simulink model "AllModes"  (R2022a)
settings: Solver=FixedStepAuto  StartTime=0.0  StopTime=10.0  FixedStep=1e-3  RelTol=1e-3  EnableMultiTasking=on
undefined symbols (not defined in the file): D0, D1, D10, D11, D12, D13, D2, D3, D4, D5, D6, D7, D8, D9, PTA0, PTA1, PTA2, PTB23, PTB9, PTC16, PTC17, PTC2, PTC3, PTC4, PTD0, PTD1, PTD2, PTD3
libraries: frdmk64flib x14
settings Model: ExtModeTrigDuration=5  Creator=bmile  LastModifiedBy=Motz
settings OptimizationCC: EnhancedBackFolding=on  PassReuseOutputArgsAs=Individual arguments  ZeroExternalMemoryAtStartup=off  ZeroInternalMemoryAtStartup=off  MaxStackSize=64  OptimizeBlockOrder=speed  DifferentSizesBufferReuse=on  OptimizationCustomize=off  EfficientTunableParamExpr=on
settings DebuggingCC: ParameterTunabilityLossMsg=error
settings HardwareCC: ProdBitPerPointer=32  ProdBitPerSizeT=32  ProdBitPerPtrDiffT=32  ProdLargestAtomicInteger=Long  ProdLargestAtomicFloat=Double  ProdWordSize=32  ProdHWDeviceType=ARM Compatible->ARM Cortex
settings SFSimCC: MATLABDynamicMemAlloc=off
settings RTWCC: SystemTargetFile=ert.tlc  HardwareBoard=NXP FRDM-K64F  TLCOptions="-aInlineSetEventsForThisBaseRateFcn=TLC_FALSE -aSuppressMultiTaskScheduler=TLC_FALSE  -aRateBasedStepFcn=0"  TemplateMakefile=ert_default_tmf  Toolchain=GNU Tools for ARM Embedded Processors
settings CodeAppCC: ForceParamTrailComments=on  IgnoreCustomStorageClasses=off  OperatorAnnotations=on  SimulinkDataObjDesc=on  SFDataObjDesc=on  InsertBlockDesc=on
settings ERTTargetCC: ExtModeTransport=4  ExtModeMexFile=sendToCommService

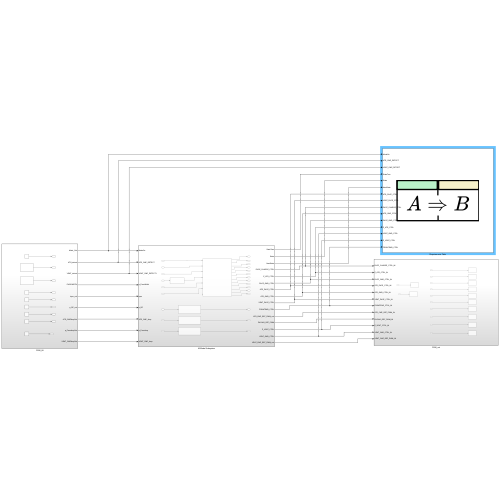
[thumbnail: Simulink's stored preview of the top-level diagram]
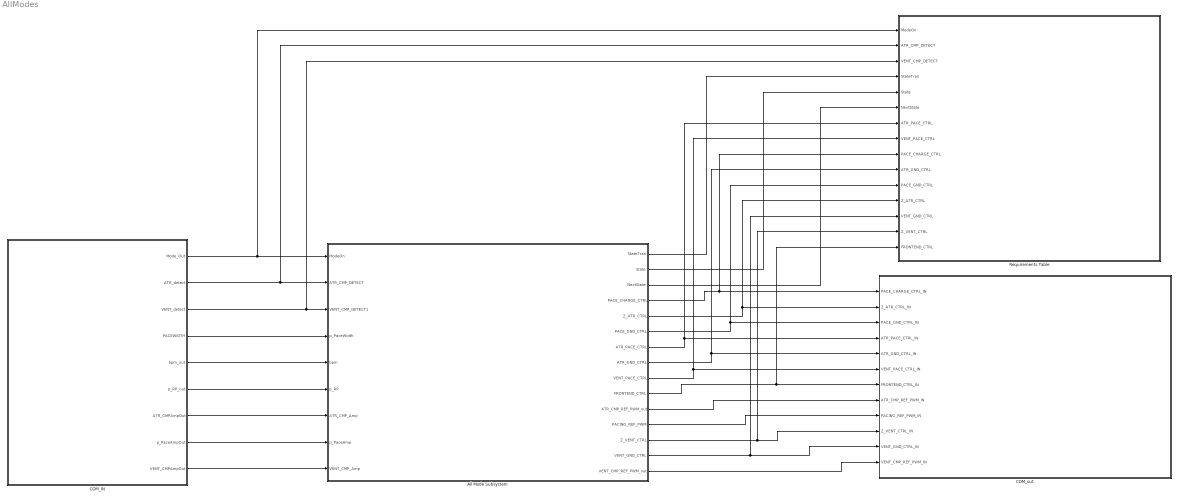
== system AllModes ==
  All Mode Subsystem : Subsystem
  COM_IN : Subsystem
  COM_out : Subsystem
  Requirements Table : Requirements Table  TreatAsAtomicUnit=on
  wires:
  COM_IN/1(Mode_Out) -> All Mode Subsystem/1(ModeOn), Requirements Table/1(ModeOn)
  COM_IN/4(PACEWIDTH) -> All Mode Subsystem/4(p_PaceWidth)
  COM_IN/5(bpm_out) -> All Mode Subsystem/5(bpm)
  COM_IN/6(p_RP_out) -> All Mode Subsystem/6(p_RP)
  COM_IN/7(ATR_CMPAmpOut) -> All Mode Subsystem/7(ATR_CMP_Amp)
  COM_IN/8(p_PaceAmpOut) -> All Mode Subsystem/8(p_PaceAmp)
  COM_IN/9(VENT_CMPAmpOut) -> All Mode Subsystem/9(VENT_CMP_Amp)
  All Mode Subsystem/4(PACE_CHARGE_CTRL) -> Requirements Table/9(PACE_CHARGE_CTRL), COM_out/1(PACE_CHARGE_CTRL_IN)
  All Mode Subsystem/5(Z_ATR_CTRL) -> Requirements Table/12(Z_ATR_CTRL), COM_out/2(Z_ATR_CTRL_IN)
  All Mode Subsystem/6(PACE_GND_CTRL) -> Requirements Table/11(PACE_GND_CTRL), COM_out/3(PACE_GND_CTRL_IN)
  All Mode Subsystem/7(ATR_PACE_CTRL) -> Requirements Table/7(ATR_PACE_CTRL), COM_out/4(ATR_PACE_CTRL_IN)
  All Mode Subsystem/9(VENT_PACE_CTRL) -> Requirements Table/8(VENT_PACE_CTRL), COM_out/6(VENT_PACE_CTRL_IN)
  All Mode Subsystem/10(FRONTEND_CTRL) -> Requirements Table/15(FRONTEND_CTRL), COM_out/7(FRONTEND_CTRL_IN)
  All Mode Subsystem/11(ATR_CMP_REF_PWM_out) -> COM_out/8(ATR_CMP_REF_PWM_IN)
  All Mode Subsystem/12(PACING_REF_PWM) -> COM_out/9(PACING_REF_PWM_IN)
  All Mode Subsystem/13(Z_VENT_CTRL) -> Requirements Table/14(Z_VENT_CTRL), COM_out/10(Z_VENT_CTRL_IN)
  All Mode Subsystem/14(VENT_GND_CTRL) -> Requirements Table/13(VENT_GND_CTRL), COM_out/11(VENT_GND_CTRL_IN)
  All Mode Subsystem/15(VENT_CMP_REF_PWM_out) -> COM_out/12(VENT_CMP_REF_PWM_IN)
  All Mode Subsystem/3(NextState) -> Requirements Table/6(NextState)
  All Mode Subsystem/2(State) -> Requirements Table/5(State)
  All Mode Subsystem/8(ATR_GND_CTRL) -> Requirements Table/10(ATR_GND_CTRL), COM_out/5(ATR_GND_CTRL_IN)
  All Mode Subsystem/1(StateTran) -> Requirements Table/4(StateTran)
  COM_IN/2(ATR_detect) -> All Mode Subsystem/2(ATR_CMP_DETECT), Requirements Table/2(ATR_CMP_DETECT)
  COM_IN/3(VENT_detect) -> Requirements Table/3(VENT_CMP_DETECT), All Mode Subsystem/3(VENT_CMP_DETECT1)

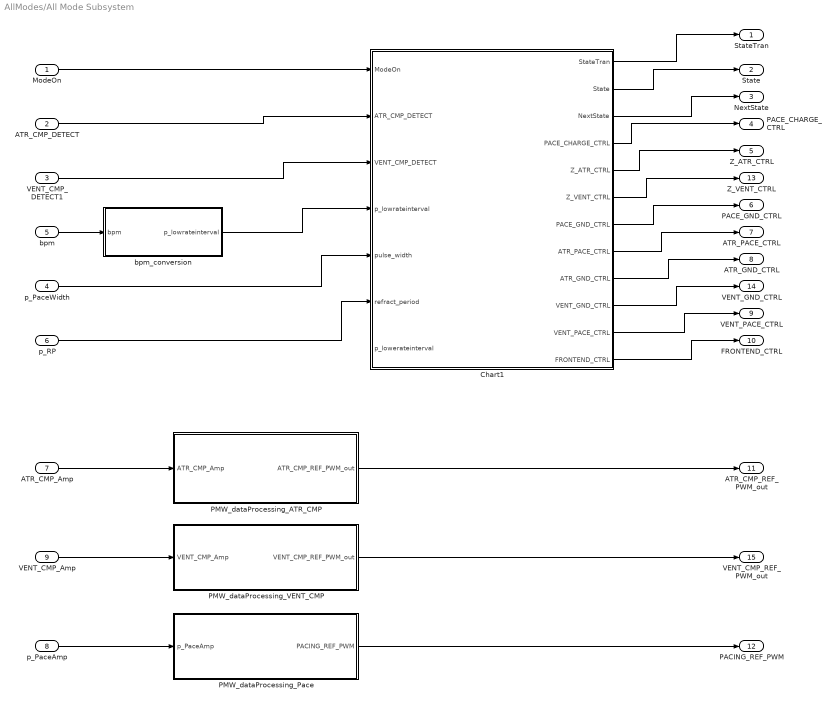
== system AllModes/All Mode Subsystem ==
  ModeOn : Inport
  ATR_CMP_DETECT : Inport  Port=2
  VENT_CMP_DETECT1 : Inport  Port=3
  p_PaceWidth : Inport  Port=4
  bpm : Inport  Port=5
  p_RP : Inport  Port=6
  ATR_CMP_Amp : Inport  Port=7
  p_PaceAmp : Inport  Port=8
  VENT_CMP_Amp : Inport  Port=9
  Chart1 : Stateflow chart  TreatAsAtomicUnit=on
      settings: PortSchema="{\"entries\":[{\"content\":{\"sides\":[{\"content\":{\"connectorIds\":[\"In1\",\"In2\",\"In3\",\"In4\",\"In5\",\"In6\",\"In7\"]},\"type\":\"ConnectorPlacement.EquallySpacedRectSide\",\"uuid\":\"7ea964f2-2529-4e69-b20d-c2fa6008c3a7\"},{\"content\":{\"connectorIds\":[\"Out12\",\"Out1\",\"Out11\",\"Out2\",\"Out3\",\"Out4\",\"Out5\",\"Out6\",\"Out7\",\"Out8\",\"Out9\",\"Out10\"],\"side\":\"RIGHT\"},\"type\":\"ConnectorPlacement.EquallySpacedRectSide\",\"uuid\":\"c561387b-bc02-43ab-893b-c9cb757a1c6a\"},{\"content\":{\"connectorIds\":[],\"side\":\"TOP\"},\"type\":\"ConnectorPlacement.EquallySpacedRectSide\",\"uuid\":\"1f667392-9a0f-4cad-82e3-6fe4d50b6af4\"}]},\"type\":\"ConnectorPlacement.EquallySpacedConnector\",\"uuid\":\"bd362c40-ffc0-452d-8626-3f1602423ca2\"}],\"packageUris\":[\"http://schema.mathworks.com/mf0/Connector/R2020b\"],\"version\":\"1.0\"}"
  PMW_dataProcessing_ATR_CMP : Subsystem
  PMW_dataProcessing_Pace : Subsystem
  PMW_dataProcessing_VENT_CMP : Subsystem
  bpm_conversion : Subsystem
  StateTran : Outport
  State : Outport  Port=2
  NextState : Outport  Port=3
  PACE_CHARGE_CTRL : Outport  Port=4
  Z_ATR_CTRL : Outport  Port=5
  PACE_GND_CTRL : Outport  Port=6
  ATR_PACE_CTRL : Outport  Port=7
  ATR_GND_CTRL : Outport  Port=8
  VENT_PACE_CTRL : Outport  Port=9
  FRONTEND_CTRL : Outport  Port=10
  ATR_CMP_REF_PWM_out : Outport  Port=11
  PACING_REF_PWM : Outport  Port=12
  Z_VENT_CTRL : Outport  Port=13
  VENT_GND_CTRL : Outport  Port=14
  VENT_CMP_REF_PWM_out : Outport  Port=15
  wires:
  Chart1/10(FRONTEND_CTRL) -> FRONTEND_CTRL/1
  Chart1/9(VENT_PACE_CTRL) -> VENT_PACE_CTRL/1
  Chart1/7(ATR_GND_CTRL) -> ATR_GND_CTRL/1
  Chart1/6(ATR_PACE_CTRL) -> ATR_PACE_CTRL/1
  Chart1/5(PACE_GND_CTRL) -> PACE_GND_CTRL/1
  Chart1/3(Z_ATR_CTRL) -> Z_ATR_CTRL/1
  Chart1/2(PACE_CHARGE_CTRL) -> PACE_CHARGE_CTRL/1
  p_RP/1 -> Chart1/6(refract_period)
  p_PaceWidth/1 -> Chart1/5(pulse_width)
  ATR_CMP_DETECT/1 -> Chart1/2(ATR_CMP_DETECT)
  Chart1/1(State) -> State/1
  ModeOn/1 -> Chart1/1(ModeOn)
  Chart1/4(Z_VENT_CTRL) -> Z_VENT_CTRL/1
  Chart1/8(VENT_GND_CTRL) -> VENT_GND_CTRL/1
  VENT_CMP_DETECT1/1 -> Chart1/3(VENT_CMP_DETECT)
  ATR_CMP_Amp/1 -> PMW_dataProcessing_ATR_CMP/1(ATR_CMP_Amp)
  p_PaceAmp/1 -> PMW_dataProcessing_Pace/1(p_PaceAmp)
  VENT_CMP_Amp/1 -> PMW_dataProcessing_VENT_CMP/1(VENT_CMP_Amp)
  PMW_dataProcessing_Pace/1(PACING_REF_PWM) -> PACING_REF_PWM/1
  PMW_dataProcessing_VENT_CMP/1(VENT_CMP_REF_PWM_out) -> VENT_CMP_REF_PWM_out/1
  PMW_dataProcessing_ATR_CMP/1(ATR_CMP_REF_PWM_out) -> ATR_CMP_REF_PWM_out/1
  bpm/1 -> bpm_conversion/1(bpm)
  bpm_conversion/1(p_lowrateinterval) -> Chart1/4(p_lowrateinterval)
  Chart1/11(NextState) -> NextState/1
  Chart1/12(StateTran) -> StateTran/1

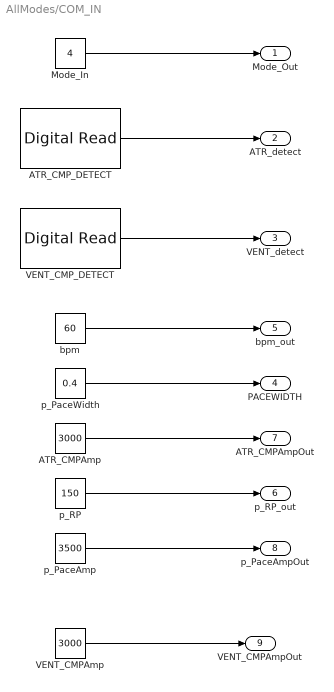
== system AllModes/COM_IN ==
  ATR_CMPAmp : Constant  Value=3000
  ATR_CMP_DETECT : frdmk64flib/Digital Read  Whichpin=PTC16 (D0)  SampleTime=-1
  Mode_In : Constant  Value=4
  VENT_CMPAmp : Constant  Value=3000
  VENT_CMP_DETECT : frdmk64flib/Digital Read  Whichpin=PTC17 (D1)  SampleTime=-1
  bpm : Constant  Value=60
  p_PaceAmp : Constant  Value=3500
  p_PaceWidth : Constant  Value=0.4
  p_RP : Constant  Value=150
  Mode_Out : Outport
  ATR_detect : Outport  Port=2
  VENT_detect : Outport  Port=3
  PACEWIDTH : Outport  Port=4
  bpm_out : Outport  Port=5
  p_RP_out : Outport  Port=6
  ATR_CMPAmpOut : Outport  Port=7
  p_PaceAmpOut : Outport  Port=8
  VENT_CMPAmpOut : Outport  Port=9
  wires:
  Mode_In/1 -> Mode_Out/1
  ATR_CMP_DETECT/1 -> ATR_detect/1
  bpm/1 -> bpm_out/1
  ATR_CMPAmp/1 -> ATR_CMPAmpOut/1
  VENT_CMP_DETECT/1 -> VENT_detect/1
  p_PaceWidth/1 -> PACEWIDTH/1
  p_RP/1 -> p_RP_out/1
  p_PaceAmp/1 -> p_PaceAmpOut/1
  VENT_CMPAmp/1 -> VENT_CMPAmpOut/1

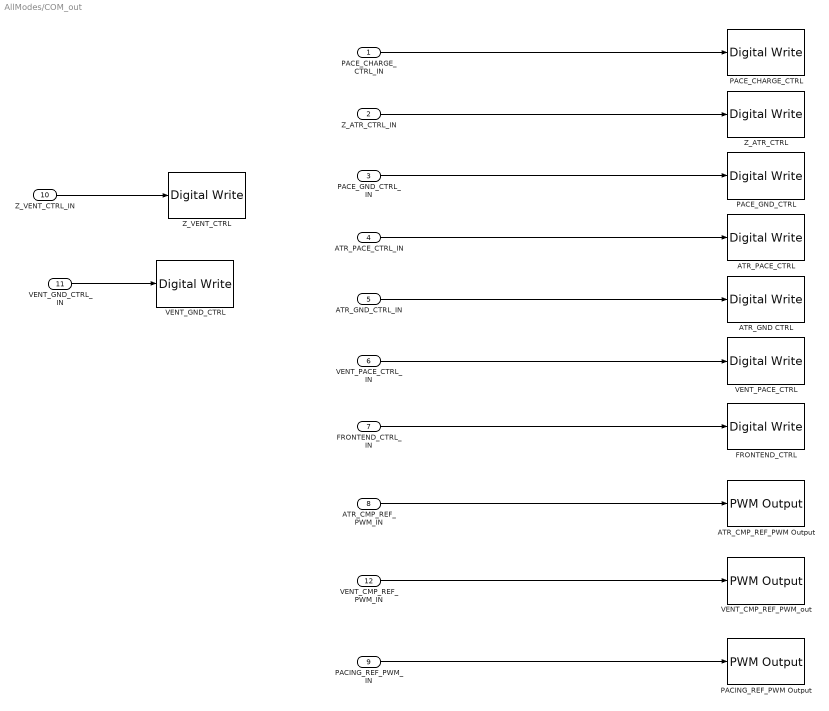
== system AllModes/COM_out ==
  PACE_CHARGE_CTRL_IN : Inport
  Z_ATR_CTRL_IN : Inport  Port=2
  PACE_GND_CTRL_IN : Inport  Port=3
  ATR_PACE_CTRL_IN : Inport  Port=4
  ATR_GND_CTRL_IN : Inport  Port=5
  VENT_PACE_CTRL_IN : Inport  Port=6
  FRONTEND_CTRL_IN : Inport  Port=7
  ATR_CMP_REF_PWM_IN : Inport  Port=8
  PACING_REF_PWM_IN : Inport  Port=9
  Z_VENT_CTRL_IN : Inport  Port=10
  VENT_GND_CTRL_IN : Inport  Port=11
  VENT_CMP_REF_PWM_IN : Inport  Port=12
  ATR_CMP_REF_PWM Output : frdmk64flib/PWM Output  Whichpin=PTC2 (D6)  InitialFrequency=2000  InitialDutyCycle=0
  ATR_GND CTRL : frdmk64flib/Digital Write  Whichpin=PTD2 (D11)
  ATR_PACE_CTRL : frdmk64flib/Digital Write  Whichpin=PTA0 (D8)
  FRONTEND_CTRL : frdmk64flib/Digital Write  Whichpin=PTD1 (D13)
  PACE_CHARGE_CTRL : frdmk64flib/Digital Write  Whichpin=PTB9 (D2)
  PACE_GND_CTRL : frdmk64flib/Digital Write  Whichpin=PTD0 (D10)
  PACING_REF_PWM Output : frdmk64flib/PWM Output  Whichpin=PTA2 (D5)  InitialFrequency=2000  InitialDutyCycle=0
  VENT_CMP_REF_PWM_out : frdmk64flib/PWM Output  Whichpin=PTA1 (D3)  InitialFrequency=2000  InitialDutyCycle=0
  VENT_GND_CTRL : frdmk64flib/Digital Write  Whichpin=PTD3 (D12)
  VENT_PACE_CTRL : frdmk64flib/Digital Write  Whichpin=PTC4 (D9)
  Z_ATR_CTRL : frdmk64flib/Digital Write  Whichpin=PTB23 (D4)
  Z_VENT_CTRL : frdmk64flib/Digital Write  Whichpin=PTC3 (D7)
  wires:
  PACE_CHARGE_CTRL_IN/1 -> PACE_CHARGE_CTRL/1
  PACE_GND_CTRL_IN/1 -> PACE_GND_CTRL/1
  Z_ATR_CTRL_IN/1 -> Z_ATR_CTRL/1
  ATR_PACE_CTRL_IN/1 -> ATR_PACE_CTRL/1
  ATR_GND_CTRL_IN/1 -> ATR_GND CTRL/1
  VENT_PACE_CTRL_IN/1 -> VENT_PACE_CTRL/1
  FRONTEND_CTRL_IN/1 -> FRONTEND_CTRL/1
  PACING_REF_PWM_IN/1 -> PACING_REF_PWM Output/1
  ATR_CMP_REF_PWM_IN/1 -> ATR_CMP_REF_PWM Output/1
  VENT_GND_CTRL_IN/1 -> VENT_GND_CTRL/1
  Z_VENT_CTRL_IN/1 -> Z_VENT_CTRL/1
  VENT_CMP_REF_PWM_IN/1 -> VENT_CMP_REF_PWM_out/1

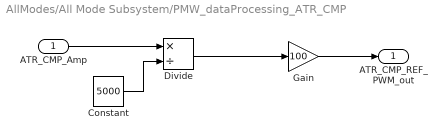
== system AllModes/All Mode Subsystem/PMW_dataProcessing_ATR_CMP ==
  ATR_CMP_Amp : Inport
  Constant : Constant  Value=5000
  Divide : Product  Inputs=*/
  Gain : Gain  Gain=100
  ATR_CMP_REF_PWM_out : Outport
  wires:
  Divide/1 -> Gain/1
  Constant/1 -> Divide/2
  ATR_CMP_Amp/1 -> Divide/1
  Gain/1 -> ATR_CMP_REF_PWM_out/1

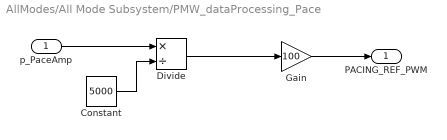
== system AllModes/All Mode Subsystem/PMW_dataProcessing_Pace ==
  p_PaceAmp : Inport
  Constant : Constant  Value=5000
  Divide : Product  Inputs=*/
  Gain : Gain  Gain=100
  PACING_REF_PWM : Outport
  wires:
  Divide/1 -> Gain/1
  Constant/1 -> Divide/2
  p_PaceAmp/1 -> Divide/1
  Gain/1 -> PACING_REF_PWM/1

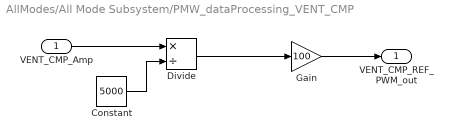
== system AllModes/All Mode Subsystem/PMW_dataProcessing_VENT_CMP ==
  VENT_CMP_Amp : Inport
  Constant : Constant  Value=5000
  Divide : Product  Inputs=*/
  Gain : Gain  Gain=100
  VENT_CMP_REF_PWM_out : Outport
  wires:
  Divide/1 -> Gain/1
  Constant/1 -> Divide/2
  VENT_CMP_Amp/1 -> Divide/1
  Gain/1 -> VENT_CMP_REF_PWM_out/1

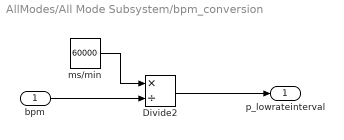
== system AllModes/All Mode Subsystem/bpm_conversion ==
  bpm : Inport
  Divide2 : Product  Inputs=*/
  ms/min : Constant  Value=60000
  p_lowrateinterval : Outport
  wires:
  ms/min/1 -> Divide2/1
  bpm/1 -> Divide2/2
  Divide2/1 -> p_lowrateinterval/1

== stateflow chart AllModes/Requirements Table ==
  (default) -> (junction 1073742992)
  (junction 1073742992) -> (junction 1073742993) : {
      | % SF_REQ_REV_07
      | }
  (junction 1073742993) -> (junction 1073742995) : {
      | % HEADER_ASSIGNMENTS
      |
      | }
  (junction 1073742995) -> (junction 1073742997) : {
      | % START_A_4
      | }
  (junction 1073742997) -> (junction 1073742999) : {
      | }
  (junction 1073742999) -> (junction 1073743001)
  (junction 1073743001) -> (junction 1073743003) : {
      | }
  (junction 1073743003) -> (junction 1073743005) : {
      | % END_A_4
      | }
  (junction 1073743005) -> (junction 1073743007) : {
      | % START_R_7
      | }
  (junction 1073743007) -> (junction 1073743009) : {
      | }
  (junction 1073743009) -> (junction 1073743011)
  (junction 1073743011) -> (junction 1073743013) [order 1] : [(((State) == (0)))]
  (junction 1073743011) -> (junction 1073743091) [order 2]
  (junction 1073743013) -> (junction 1073743015) : {
      | reqtable_postcondition((((NextState) == (0))) && (((ATR_PACE_CTRL) == (false))) && (((VENT_PACE_CTRL) == (false))) && (((PACE_CHARGE_CTRL) == (false))) && (((ATR_GND_CTRL) == (false))) && (((PACE_GND_CTRL) == (false))) && (((Z_ATR_CTRL) == (false))) && (((VENT_GND_CTRL) == (false))) && (((Z_VENT_CTRL) == (false))) && (((FRONTEND_CTRL) == (false))), 'R:1');
      |
      |
      | }
  (junction 1073743015) -> (junction 1073743017) : {
      | }
  (junction 1073743017) -> (junction 1073743019) : {
      | % START_R_10
      | }
  (junction 1073743019) -> (junction 1073743021) : {
      | }
  (junction 1073743021) -> (junction 1073743023)
  (junction 1073743023) -> (junction 1073743025) [order 1] : [(((StateTran) == (true))) && (((ModeOn) == (1)))]
  (junction 1073743023) -> (junction 1073743031) [order 2]
  (junction 1073743025) -> (junction 1073743027) : {
      | reqtable_postcondition((((NextState) == (1))) && (((ATR_PACE_CTRL) == (false))) && (((VENT_PACE_CTRL) == (false))) && (((PACE_CHARGE_CTRL) == (false))) && (((ATR_GND_CTRL) == (false))) && (((PACE_GND_CTRL) == (false))) && (((Z_ATR_CTRL) == (false))) && (((VENT_GND_CTRL) == (false))) && (((Z_VENT_CTRL) == (false))) && (((FRONTEND_CTRL) == (false))), 'R:1.1');
      |
      |
      | }
  (junction 1073743027) -> (junction 1073743029) : {
      | }
  (junction 1073743029) -> (junction 1073743031)
  (junction 1073743031) -> (junction 1073743033)
  (junction 1073743033) -> (junction 1073743035) : {
      | % END_R_10
      | }
  (junction 1073743035) -> (junction 1073743037) : {
      | % START_R_16
      | }
  (junction 1073743037) -> (junction 1073743039) : {
      | }
  (junction 1073743039) -> (junction 1073743041)
  (junction 1073743041) -> (junction 1073743043) [order 1] : [(((StateTran) == (true))) && (((ModeOn) == (2)))]
  (junction 1073743041) -> (junction 1073743049) [order 2]
  (junction 1073743043) -> (junction 1073743045) : {
      | reqtable_postcondition((((NextState) == (2))) && (((ATR_PACE_CTRL) == (false))) && (((VENT_PACE_CTRL) == (false))) && (((PACE_CHARGE_CTRL) == (false))) && (((ATR_GND_CTRL) == (false))) && (((PACE_GND_CTRL) == (false))) && (((Z_ATR_CTRL) == (false))) && (((VENT_GND_CTRL) == (false))) && (((Z_VENT_CTRL) == (false))) && (((FRONTEND_CTRL) == (false))), 'R:1.2');
      |
      |
      | }
  (junction 1073743045) -> (junction 1073743047) : {
      | }
  (junction 1073743047) -> (junction 1073743049)
  (junction 1073743049) -> (junction 1073743051)
  (junction 1073743051) -> (junction 1073743053) : {
      | % END_R_16
      | }
  (junction 1073743053) -> (junction 1073743055) : {
      | % START_R_19
      | }
  (junction 1073743055) -> (junction 1073743057) : {
      | }
  (junction 1073743057) -> (junction 1073743059)
  (junction 1073743059) -> (junction 1073743061) [order 1] : [(((StateTran) == (true))) && (((ModeOn) == (3)))]
  (junction 1073743059) -> (junction 1073743067) [order 2]
  (junction 1073743061) -> (junction 1073743063) : {
      | reqtable_postcondition((((NextState) == (3))) && (((ATR_PACE_CTRL) == (false))) && (((VENT_PACE_CTRL) == (false))) && (((PACE_CHARGE_CTRL) == (false))) && (((ATR_GND_CTRL) == (false))) && (((PACE_GND_CTRL) == (false))) && (((Z_ATR_CTRL) == (false))) && (((VENT_GND_CTRL) == (false))) && (((Z_VENT_CTRL) == (false))) && (((FRONTEND_CTRL) == (false))), 'R:1.3');
      |
      |
      | }
  (junction 1073743063) -> (junction 1073743065) : {
      | }
  (junction 1073743065) -> (junction 1073743067)
  (junction 1073743067) -> (junction 1073743069)
  (junction 1073743069) -> (junction 1073743071) : {
      | % END_R_19
      | }
  (junction 1073743071) -> (junction 1073743073) : {
      | % START_R_22
      | }
  (junction 1073743073) -> (junction 1073743075) : {
      | }
  (junction 1073743075) -> (junction 1073743077)
  (junction 1073743077) -> (junction 1073743079) [order 1] : [(((StateTran) == (true))) && (((ModeOn) == (4)))]
  (junction 1073743077) -> (junction 1073743085) [order 2]
  (junction 1073743079) -> (junction 1073743081) : {
      | reqtable_postcondition((((NextState) == (4))), 'R:1.4');
      |
      |
      | }
  (junction 1073743081) -> (junction 1073743083) : {
      | }
  (junction 1073743083) -> (junction 1073743085)
  (junction 1073743085) -> (junction 1073743087)
  (junction 1073743087) -> (junction 1073743089) : {
      | % END_R_22
      | }
  (junction 1073743089) -> (junction 1073743091)
  (junction 1073743091) -> (junction 1073743093)
  (junction 1073743093) -> (junction 1073743095) : {
      | % END_R_7
      | }
  (junction 1073743095) -> (junction 1073743097) : {
      | % START_R_1
      | }
  (junction 1073743097) -> (junction 1073743099) : {
      | }
  (junction 1073743099) -> (junction 1073743101)
  (junction 1073743101) -> (junction 1073743103) [order 1] : [(((State) == (1)))]
  (junction 1073743101) -> (junction 1073743127) [order 2]
  (junction 1073743103) -> (junction 1073743105) : {
      | reqtable_postcondition((((NextState) == (0))) && (((ATR_PACE_CTRL) == (false))) && (((VENT_PACE_CTRL) == (false))) && (((PACE_CHARGE_CTRL) == (true))) && (((ATR_GND_CTRL) == (true))) && (((PACE_GND_CTRL) == (true))) && (((Z_ATR_CTRL) == (false))) && (((VENT_GND_CTRL) == (false))) && (((Z_VENT_CTRL) == (false))) && (((FRONTEND_CTRL) == (false))), 'R:2');
      |
      |
      | }
  (junction 1073743105) -> (junction 1073743107) : {
      | }
  (junction 1073743107) -> (junction 1073743109) : {
      | % START_R_28
      | }
  (junction 1073743109) -> (junction 1073743111) : {
      | }
  (junction 1073743111) -> (junction 1073743113)
  (junction 1073743113) -> (junction 1073743115) [order 1] : [(((StateTran) == (true)))]
  (junction 1073743113) -> (junction 1073743121) [order 2]
  (junction 1073743115) -> (junction 1073743117) : {
      | reqtable_postcondition((((NextState) == (2))), 'R:2.1');
      |
      |
      | }
  (junction 1073743117) -> (junction 1073743119) : {
      | }
  (junction 1073743119) -> (junction 1073743121)
  (junction 1073743121) -> (junction 1073743123)
  (junction 1073743123) -> (junction 1073743125) : {
      | % END_R_28
      | }
  (junction 1073743125) -> (junction 1073743127)
  (junction 1073743127) -> (junction 1073743129)
  (junction 1073743129) -> (junction 1073743131) : {
      | % END_R_1
      | }
  (junction 1073743131) -> (junction 1073743133) : {
      | % START_R_25
      | }
  (junction 1073743133) -> (junction 1073743135) : {
      | }
  (junction 1073743135) -> (junction 1073743137)
  (junction 1073743137) -> (junction 1073743139) [order 1] : [(((State) == (2)))]
  (junction 1073743137) -> (junction 1073743313) [order 2]
  (junction 1073743139) -> (junction 1073743141) : {
      | reqtable_postcondition((((NextState) == (0))) && (((ATR_PACE_CTRL) == (true))) && (((VENT_PACE_CTRL) == (false))) && (((PACE_CHARGE_CTRL) == (false))) && (((ATR_GND_CTRL) == (false))) && (((PACE_GND_CTRL) == (true))) && (((Z_ATR_CTRL) == (false))) && (((VENT_GND_CTRL) == (false))) && (((Z_VENT_CTRL) == (false))) && (((FRONTEND_CTRL) == (false))), 'R:3');
      |
      |
      | }
  (junction 1073743141) -> (junction 1073743143) : {
      | }
  (junction 1073743143) -> (junction 1073743145) : {
      | % START_R_31
      | }
  (junction 1073743145) -> (junction 1073743147) : {
      | }
  (junction 1073743147) -> (junction 1073743149)
  (junction 1073743149) -> (junction 1073743151) [order 1] : [(((StateTran) == (true)))]
  (junction 1073743149) -> (junction 1073743157) [order 2]
  (junction 1073743151) -> (junction 1073743153) : {
      | reqtable_postcondition((((NextState) == (1))), 'R:3.1');
      |
      |
      | }
  (junction 1073743153) -> (junction 1073743155) : {
      | }
  (junction 1073743155) -> (junction 1073743157)
  (junction 1073743157) -> (junction 1073743159)
  (junction 1073743159) -> (junction 1073744214) : {
      | % END_R_31
      | }
  (junction 1073744214) -> (junction 1073743313)
  (junction 1073743313) -> (junction 1073743315)
  (junction 1073743315) -> (junction 1073743317) : {
      | % END_R_25
      | }
  (junction 1073743317) -> (junction 1073744220) : {
      | % START_R_34
      | }
  (junction 1073744220) -> (junction 1073744222) : {
      | }
  (junction 1073744222) -> (junction 1073744224)
  (junction 1073744224) -> (junction 1073744226) [order 1] : [(((State) == (3)))]
  (junction 1073744224) -> (junction 1073744250) [order 2]
  (junction 1073744226) -> (junction 1073744228) : {
      | reqtable_postcondition((((NextState) == (0))) && (((ATR_PACE_CTRL) == (false))) && (((VENT_PACE_CTRL) == (false))) && (((PACE_CHARGE_CTRL) == (true))) && (((ATR_GND_CTRL) == (false))) && (((PACE_GND_CTRL) == (true))) && (((Z_ATR_CTRL) == (false))) && (((VENT_GND_CTRL) == (true))) && (((Z_VENT_CTRL) == (false))) && (((FRONTEND_CTRL) == (false))), 'R:4');
      |
      |
      | }
  (junction 1073744228) -> (junction 1073744230) : {
      | }
  (junction 1073744230) -> (junction 1073744232) : {
      | % START_R_37
      | }
  (junction 1073744232) -> (junction 1073744234) : {
      | }
  (junction 1073744234) -> (junction 1073744236)
  (junction 1073744236) -> (junction 1073744238) [order 1] : [(((StateTran) == (true)))]
  (junction 1073744236) -> (junction 1073744244) [order 2]
  (junction 1073744238) -> (junction 1073744240) : {
      | reqtable_postcondition((((NextState) == (4))), 'R:4.1');
      |
      |
      | }
  (junction 1073744240) -> (junction 1073744242) : {
      | }
  (junction 1073744242) -> (junction 1073744244)
  (junction 1073744244) -> (junction 1073744246)
  (junction 1073744246) -> (junction 1073744248) : {
      | % END_R_37
      | }
  (junction 1073744248) -> (junction 1073744250)
  (junction 1073744250) -> (junction 1073744252)
  (junction 1073744252) -> (junction 1073744254) : {
      | % END_R_34
      | }
  (junction 1073744254) -> (junction 1073744260) : {
      | % START_R_43
      | }
  (junction 1073744260) -> (junction 1073744262) : {
      | }
  (junction 1073744262) -> (junction 1073744264)
  (junction 1073744264) -> (junction 1073744266) [order 1] : [(((State) == (4)))]
  (junction 1073744264) -> (junction 1073744290) [order 2]
  (junction 1073744266) -> (junction 1073744268) : {
      | reqtable_postcondition((((NextState) == (0))) && (((ATR_PACE_CTRL) == (false))) && (((VENT_PACE_CTRL) == (true))) && (((PACE_CHARGE_CTRL) == (false))) && (((ATR_GND_CTRL) == (false))) && (((PACE_GND_CTRL) == (true))) && (((Z_ATR_CTRL) == (false))) && (((VENT_GND_CTRL) == (false))) && (((Z_VENT_CTRL) == (false))) && (((FRONTEND_CTRL) == (false))), 'R:5');
      |
      |
      | }
  (junction 1073744268) -> (junction 1073744270) : {
      | }
  (junction 1073744270) -> (junction 1073744272) : {
      | % START_R_46
      | }
  (junction 1073744272) -> (junction 1073744274) : {
      | }
  (junction 1073744274) -> (junction 1073744276)
  (junction 1073744276) -> (junction 1073744278) [order 1] : [(((StateTran) == (true)))]
  (junction 1073744276) -> (junction 1073744284) [order 2]
  (junction 1073744278) -> (junction 1073744280) : {
      | reqtable_postcondition((((NextState) == (3))), 'R:5.1');
      |
      |
      | }
  (junction 1073744280) -> (junction 1073744282) : {
      | }
  (junction 1073744282) -> (junction 1073744284)
  (junction 1073744284) -> (junction 1073744286)
  (junction 1073744286) -> (junction 1073744288) : {
      | % END_R_46
      | }
  (junction 1073744288) -> (junction 1073744290)
  (junction 1073744290) -> (junction 1073744292)
  (junction 1073744292) -> (junction 1073744294) : {
      | % END_R_43
      | }
  (junction 1073744294) -> (junction 1073744121) : {
      | % START_R_49
      | }
  (junction 1073744121) -> (junction 1073744123) : {
      | }
  (junction 1073744123) -> (junction 1073744125)
  (junction 1073744125) -> (junction 1073744127) [order 1] : [(((State) == (5)))]
  (junction 1073744125) -> (junction 1073744169) [order 2]
  (junction 1073744127) -> (junction 1073744129) : {
      | reqtable_postcondition((((NextState) == (0))) && (((ATR_PACE_CTRL) == (false))) && (((VENT_PACE_CTRL) == (false))) && (((PACE_CHARGE_CTRL) == (true))) && (((ATR_GND_CTRL) == (true))) && (((PACE_GND_CTRL) == (true))) && (((Z_ATR_CTRL) == (false))) && (((VENT_GND_CTRL) == (false))) && (((Z_VENT_CTRL) == (false))) && (((FRONTEND_CTRL) == (true))), 'R:6');
      |
      |
      | }
  (junction 1073744129) -> (junction 1073744131) : {
      | }
  (junction 1073744131) -> (junction 1073744133) : {
      | % START_R_58
      | }
  (junction 1073744133) -> (junction 1073744135) : {
      | }
  (junction 1073744135) -> (junction 1073744137)
  (junction 1073744137) -> (junction 1073744139) [order 1] : [(((StateTran) == (true))) && (((ATR_CMP_DETECT) == (true)))]
  (junction 1073744137) -> (junction 1073744145) [order 2]
  (junction 1073744139) -> (junction 1073744141) : {
      | reqtable_postcondition((((NextState) == (6))), 'R:6.1');
      |
      |
      | }
  (junction 1073744141) -> (junction 1073744143) : {
      | }
  (junction 1073744143) -> (junction 1073744145)
  (junction 1073744145) -> (junction 1073744147)
  (junction 1073744147) -> (junction 1073744149) : {
      | % END_R_58
      | }
  (junction 1073744149) -> (junction 1073744151) : {
      | % START_R_67
      | }
  (junction 1073744151) -> (junction 1073744153) : {
      | }
  (junction 1073744153) -> (junction 1073744155)
  (junction 1073744155) -> (junction 1073744157) [order 1] : [(((StateTran) == (true))) && (((ATR_CMP_DETECT) == (false)))]
  (junction 1073744155) -> (junction 1073744163) [order 2]
  (junction 1073744157) -> (junction 1073744159) : {
      | reqtable_postcondition((((NextState) == (7))), 'R:6.2');
      |
      |
      | }
  (junction 1073744159) -> (junction 1073744161) : {
      | }
  (junction 1073744161) -> (junction 1073744163)
  (junction 1073744163) -> (junction 1073744165)
  (junction 1073744165) -> (junction 1073744167) : {
      | % END_R_67
      | }
  (junction 1073744167) -> (junction 1073744169)
  (junction 1073744169) -> (junction 1073744171)
  (junction 1073744171) -> (junction 1073744173) : {
      | % END_R_49
      | }
  (junction 1073744173) -> (junction 1073744081) : {
      | % START_R_52
      | }
  (junction 1073744081) -> (junction 1073744083) : {
      | }
  (junction 1073744083) -> (junction 1073744085)
  (junction 1073744085) -> (junction 1073744087) [order 1] : [(((State) == (6)))]
  (junction 1073744085) -> (junction 1073744111) [order 2]
  (junction 1073744087) -> (junction 1073744089) : {
      | reqtable_postcondition((((NextState) == (0))) && (((ATR_PACE_CTRL) == (false))) && (((VENT_PACE_CTRL) == (false))) && (((PACE_CHARGE_CTRL) == (true))) && (((ATR_GND_CTRL) == (true))) && (((PACE_GND_CTRL) == (true))) && (((Z_ATR_CTRL) == (false))) && (((VENT_GND_CTRL) == (false))) && (((Z_VENT_CTRL) == (false))) && (((FRONTEND_CTRL) == (true))), 'R:7');
      |
      |
      | }
  (junction 1073744089) -> (junction 1073744091) : {
      | }
  (junction 1073744091) -> (junction 1073744093) : {
      | % START_R_61
      | }
  (junction 1073744093) -> (junction 1073744095) : {
      | }
  (junction 1073744095) -> (junction 1073744097)
  (junction 1073744097) -> (junction 1073744099) [order 1] : [(((StateTran) == (true)))]
  (junction 1073744097) -> (junction 1073744105) [order 2]
  (junction 1073744099) -> (junction 1073744101) : {
      | reqtable_postcondition((((NextState) == (5))), 'R:7.1');
      |
      |
      | }
  (junction 1073744101) -> (junction 1073744103) : {
      | }
  (junction 1073744103) -> (junction 1073744105)
  (junction 1073744105) -> (junction 1073744107)
  (junction 1073744107) -> (junction 1073744109) : {
      | % END_R_61
      | }
  (junction 1073744109) -> (junction 1073744111)
  (junction 1073744111) -> (junction 1073744113)
  (junction 1073744113) -> (junction 1073744115) : {
      | % END_R_52
      | }
  (junction 1073744115) -> (junction 1073744041) : {
      | % START_R_55
      | }
  (junction 1073744041) -> (junction 1073744043) : {
      | }
  (junction 1073744043) -> (junction 1073744045)
  (junction 1073744045) -> (junction 1073744047) [order 1] : [(((State) == (7)))]
  (junction 1073744045) -> (junction 1073744071) [order 2]
  (junction 1073744047) -> (junction 1073744049) : {
      | reqtable_postcondition((((NextState) == (0))) && (((ATR_PACE_CTRL) == (true))) && (((VENT_PACE_CTRL) == (false))) && (((PACE_CHARGE_CTRL) == (false))) && (((ATR_GND_CTRL) == (false))) && (((PACE_GND_CTRL) == (true))) && (((Z_ATR_CTRL) == (false))) && (((VENT_GND_CTRL) == (false))) && (((Z_VENT_CTRL) == (false))) && (((FRONTEND_CTRL) == (true))), 'R:8');
      |
      |
      | }
  (junction 1073744049) -> (junction 1073744051) : {
      | }
  (junction 1073744051) -> (junction 1073744053) : {
      | % START_R_64
      | }
  (junction 1073744053) -> (junction 1073744055) : {
      | }
  (junction 1073744055) -> (junction 1073744057)
  (junction 1073744057) -> (junction 1073744059) [order 1] : [(((StateTran) == (true)))]
  (junction 1073744057) -> (junction 1073744065) [order 2]
  (junction 1073744059) -> (junction 1073744061) : {
      | reqtable_postcondition((((NextState) == (5))), 'R:8.1');
      |
      |
      | }
  (junction 1073744061) -> (junction 1073744063) : {
      | }
  (junction 1073744063) -> (junction 1073744065)
  (junction 1073744065) -> (junction 1073744067)
  (junction 1073744067) -> (junction 1073744069) : {
      | % END_R_64
      | }
  (junction 1073744069) -> (junction 1073744071)
  (junction 1073744071) -> (junction 1073744073)
  (junction 1073744073) -> (junction 1073744075) : {
      | % END_R_55
      | }
  (junction 1073744075) -> (junction 1073743982) : {
      | % START_R_70
      | }
  (junction 1073743982) -> (junction 1073743984) : {
      | }
  (junction 1073743984) -> (junction 1073743986)
  (junction 1073743986) -> (junction 1073743988) [order 1] : [(((State) == (8)))]
  (junction 1073743986) -> (junction 1073744030) [order 2]
  (junction 1073743988) -> (junction 1073743990) : {
      | reqtable_postcondition((((NextState) == (0))) && (((ATR_PACE_CTRL) == (false))) && (((VENT_PACE_CTRL) == (false))) && (((PACE_CHARGE_CTRL) == (true))) && (((ATR_GND_CTRL) == (false))) && (((PACE_GND_CTRL) == (true))) && (((Z_ATR_CTRL) == (false))) && (((VENT_GND_CTRL) == (true))) && (((Z_VENT_CTRL) == (false))) && (((FRONTEND_CTRL) == (true))), 'R:9');
      |
      |
      | }
  (junction 1073743990) -> (junction 1073743992) : {
      | }
  (junction 1073743992) -> (junction 1073743994) : {
      | % START_R_79
      | }
  (junction 1073743994) -> (junction 1073743996) : {
      | }
  (junction 1073743996) -> (junction 1073743998)
  (junction 1073743998) -> (junction 1073744000) [order 1] : [(((StateTran) == (true))) && (((VENT_CMP_DETECT) == (true)))]
  (junction 1073743998) -> (junction 1073744006) [order 2]
  (junction 1073744000) -> (junction 1073744002) : {
      | reqtable_postcondition((((NextState) == (9))), 'R:9.1');
      |
      |
      | }
  (junction 1073744002) -> (junction 1073744004) : {
      | }
  (junction 1073744004) -> (junction 1073744006)
  (junction 1073744006) -> (junction 1073744008)
  (junction 1073744008) -> (junction 1073744010) : {
      | % END_R_79
      | }
  (junction 1073744010) -> (junction 1073744012) : {
      | % START_R_82
      | }
  (junction 1073744012) -> (junction 1073744014) : {
      | }
  (junction 1073744014) -> (junction 1073744016)
  (junction 1073744016) -> (junction 1073744018) [order 1] : [(((StateTran) == (true))) && (((VENT_CMP_DETECT) == (false)))]
  (junction 1073744016) -> (junction 1073744024) [order 2]
  (junction 1073744018) -> (junction 1073744020) : {
      | reqtable_postcondition((((NextState) == (10))), 'R:9.2');
      |
      |
      | }
  (junction 1073744020) -> (junction 1073744022) : {
      | }
  (junction 1073744022) -> (junction 1073744024)
  (junction 1073744024) -> (junction 1073744026)
  (junction 1073744026) -> (junction 1073744028) : {
      | % END_R_82
      | }
  (junction 1073744028) -> (junction 1073744030)
  (junction 1073744030) -> (junction 1073744032)
  (junction 1073744032) -> (junction 1073744034) : {
      | % END_R_70
      | }
  (junction 1073744034) -> (junction 1073743942) : {
      | % START_R_73
      | }
  (junction 1073743942) -> (junction 1073743944) : {
      | }
  (junction 1073743944) -> (junction 1073743946)
  (junction 1073743946) -> (junction 1073743948) [order 1] : [(((State) == (9)))]
  (junction 1073743946) -> (junction 1073743972) [order 2]
  (junction 1073743948) -> (junction 1073743950) : {
      | reqtable_postcondition((((NextState) == (0))) && (((ATR_PACE_CTRL) == (false))) && (((VENT_PACE_CTRL) == (false))) && (((PACE_CHARGE_CTRL) == (true))) && (((ATR_GND_CTRL) == (false))) && (((PACE_GND_CTRL) == (true))) && (((Z_ATR_CTRL) == (false))) && (((VENT_GND_CTRL) == (true))) && (((Z_VENT_CTRL) == (false))) && (((FRONTEND_CTRL) == (true))), 'R:10');
      |
      |
      | }
  (junction 1073743950) -> (junction 1073743952) : {
      | }
  (junction 1073743952) -> (junction 1073743954) : {
      | % START_R_85
      | }
  (junction 1073743954) -> (junction 1073743956) : {
      | }
  (junction 1073743956) -> (junction 1073743958)
  (junction 1073743958) -> (junction 1073743960) [order 1] : [(((StateTran) == (true)))]
  (junction 1073743958) -> (junction 1073743966) [order 2]
  (junction 1073743960) -> (junction 1073743962) : {
      | reqtable_postcondition((((NextState) == (8))), 'R:10.1');
      |
      |
      | }
  (junction 1073743962) -> (junction 1073743964) : {
      | }
  (junction 1073743964) -> (junction 1073743966)
  (junction 1073743966) -> (junction 1073743968)
  (junction 1073743968) -> (junction 1073743970) : {
      | % END_R_85
      | }
  (junction 1073743970) -> (junction 1073743972)
  (junction 1073743972) -> (junction 1073743974)
  (junction 1073743974) -> (junction 1073743976) : {
      | % END_R_73
      | }
  (junction 1073743976) -> (junction 1073743902) : {
      | % START_R_76
      | }
  (junction 1073743902) -> (junction 1073743904) : {
      | }
  (junction 1073743904) -> (junction 1073743906)
  (junction 1073743906) -> (junction 1073743908) [order 1] : [(((State) == (10)))]
  (junction 1073743906) -> (junction 1073743932) [order 2]
  (junction 1073743908) -> (junction 1073743910) : {
      | reqtable_postcondition((((NextState) == (0))) && (((ATR_PACE_CTRL) == (false))) && (((VENT_PACE_CTRL) == (true))) && (((PACE_CHARGE_CTRL) == (false))) && (((ATR_GND_CTRL) == (false))) && (((PACE_GND_CTRL) == (true))) && (((Z_ATR_CTRL) == (false))) && (((VENT_GND_CTRL) == (false))) && (((Z_VENT_CTRL) == (false))) && (((FRONTEND_CTRL) == (true))), 'R:11');
      |
      |
      | }
  (junction 1073743910) -> (junction 1073743912) : {
      | }
  (junction 1073743912) -> (junction 1073743914) : {
      | % START_R_88
      | }
  (junction 1073743914) -> (junction 1073743916) : {
      | }
  (junction 1073743916) -> (junction 1073743918)
  (junction 1073743918) -> (junction 1073743920) [order 1] : [(((StateTran) == (true)))]
  (junction 1073743918) -> (junction 1073743926) [order 2]
  (junction 1073743920) -> (junction 1073743922) : {
      | reqtable_postcondition((((NextState) == (8))), 'R:11.1');
      |
      |
      | }
  (junction 1073743922) -> (junction 1073743924) : {
      | }
  (junction 1073743924) -> (junction 1073743926)
  (junction 1073743926) -> (junction 1073743928)
  (junction 1073743928) -> (junction 1073743930) : {
      | % END_R_88
      | }
  (junction 1073743930) -> (junction 1073743932)
  (junction 1073743932) -> (junction 1073743934)
  (junction 1073743934) -> (junction 1073743896) : {
      | % END_R_76
      | }
  data: ModeOn input; ATR_CMP_DETECT input; VENT_CMP_DETECT input; StateTran input; State input; NextState input; ATR_PACE_CTRL input; VENT_PACE_CTRL input; PACE_CHARGE_CTRL input; ATR_GND_CTRL input; PACE_GND_CTRL input; Z_ATR_CTRL input; VENT_GND_CTRL input; Z_VENT_CTRL input; FRONTEND_CTRL input

== stateflow chart AllModes/All Mode Subsystem/Chart1 ==
  state AOO_Charging_Discharging
    entry:
    StateTran = false
    NextState = 0
    ATR_PACE_CTRL = false
    VENT_PACE_CTRL=false
    PACE_CHARGE_CTRL = true
    ATR_GND_CTRL = true
    PACE_GND_CTRL = true
    Z_ATR_CTRL=false
    State = 1
    exit:
    StateTran = true
  state AOO_Pace_Heart
    entry:
    StateTran = false
    NextState = 0
    ATR_PACE_CTRL = true
    PACE_CHARGE_CTRL = false
    PACE_GND_CTRL = true
    ATR_GND_CTRL = false
    State = 2
    exit:
    StateTran = true
  state VOO_VENT_Charging_Discharging
    entry:
    NextState = 0
    VENT_PACE_CTRL = false
    ATR_PACE_CTRL = false
    PACE_CHARGE_CTRL = true
    VENT_GND_CTRL = true
    PACE_GND_CTRL = true
    Z_VENT_CTRL=false
    State = 3
    StateTran = false
    exit:
    StateTran = true
  state VOO_VENT_Pace_Heart
    entry:
    NextState = 0
    StateTran = false
    VENT_PACE_CTRL = true
    PACE_CHARGE_CTRL = false
    PACE_GND_CTRL = true
    VENT_GND_CTRL = false
    State = 4
    exit:
    StateTran = true
  state AAI_Pulse_Sensed
    entry:
    NextState = 0
    %FRONTEND_CTRL=false
    State = 6
    StateTran = false
    exit:
    StateTran = true
    wait_time=refract_period
  state StateOff
    %This state tells the pacemaker which
    %mode it should run, which is decided
    %by ModeOn and is checked on the
    %transistion conditions.
    entry:
    %Initialize all states to 0 or false, since
    %the pacemaker should do nothing in this
    %state.
    StateTran = false
    State = 0
    NextState = 0
    PACE_CHARGE_CTRL = false
    Z_ATR_CTRL = false
    Z_VENT_CTRL = false
    PACE_GND_CTRL = false
    ATR_PACE_CTRL = false
    ATR_GND_CTRL = false
    VENT_GND_CTRL = false
    VENT_PACE_CTRL = false
    FRONTEND_CTRL = false
    exit:
    StateTran = true
    wait_time=pulse_width
  state AAI_Charging_Discharging
    entry:
    NextState = 0
    ATR_PACE_CTRL = false
    VENT_PACE_CTRL=false
    PACE_CHARGE_CTRL = true
    ATR_GND_CTRL = true
    PACE_GND_CTRL = true
    Z_ATR_CTRL=false
    FRONTEND_CTRL=true
    State = 5
    StateTran = false
    exit:
    StateTran = true
  state AAI_Pace_Heart
    entry:
    NextState = 0
    ATR_PACE_CTRL = true
    PACE_CHARGE_CTRL = false
    PACE_GND_CTRL = true
    ATR_GND_CTRL = false
    State = 7
    StateTran = false
    exit:
    StateTran = true
    wait_time=pulse_width
  state VVI_Pulse_Sensed
    entry:
    NextState = 0
    %FRONTEND_CTRL=false
    State = 9
    StateTran = false
    exit:
    StateTran = true
    wait_time=refract_period
  state VVI_Pace_Heart
    entry:
    NextState = 0
    VENT_PACE_CTRL = true
    PACE_CHARGE_CTRL = false
    PACE_GND_CTRL = true
    VENT_GND_CTRL = false
    State = 10
    StateTran = false
    exit:
    StateTran = true
    wait_time=pulse_width
  state VVI_Charging_Discharging
    entry:
    NextState = 0
    ATR_PACE_CTRL = false
    VENT_PACE_CTRL=false
    PACE_CHARGE_CTRL = true
    VENT_GND_CTRL = true
    PACE_GND_CTRL = true
    Z_VENT_CTRL=false
    FRONTEND_CTRL=true
    State = 8
    StateTran = false
    exit:
    StateTran = true
  AOO_Charging_Discharging -> AOO_Pace_Heart : after(p_lowrateinterval-pulse_width,msec) / {NextState = 2}
  StateOff -> AOO_Charging_Discharging [order 4] : [ModeOn==1] / {NextState = 1}
  AOO_Pace_Heart -> AOO_Charging_Discharging : after(pulse_width,msec) / {NextState = 1}
  VOO_VENT_Charging_Discharging -> VOO_VENT_Pace_Heart : after(p_lowerateinterval-pulse_width,msec) / {NextState = 4}
  VOO_VENT_Pace_Heart -> VOO_VENT_Charging_Discharging : after(pulse_width,msec) / {NextState = 3}
  StateOff -> VOO_VENT_Charging_Discharging [order 3] : [ModeOn==2] / {NextState = 3}
  (default) -> StateOff
  AAI_Pulse_Sensed -> AAI_Charging_Discharging : [after(refract_period,msec)] / {NextState = 5}
  AAI_Charging_Discharging -> AAI_Pulse_Sensed [order 2] : [ATR_CMP_DETECT == 1] / {NextState = 6}
  StateOff -> AAI_Charging_Discharging [order 1] : [ModeOn==3] / {NextState = 5}
  AAI_Charging_Discharging -> AAI_Pace_Heart [order 1] : [after(p_lowrateinterval-wait_time,msec)] / {NextState = 7}
  AAI_Pace_Heart -> AAI_Charging_Discharging : after(pulse_width,msec) / {NextState = 5}
  StateOff -> VVI_Charging_Discharging [order 2] : [ModeOn==4] / {NextState = 8}
  VVI_Pulse_Sensed -> VVI_Charging_Discharging : [after(refract_period,msec)] / {NextState = 8}
  VVI_Charging_Discharging -> VVI_Pulse_Sensed [order 2] : [VENT_CMP_DETECT == 1] / {NextState = 9}
  VVI_Charging_Discharging -> VVI_Pace_Heart [order 1] : [after(p_lowrateinterval-wait_time,msec)] / {NextState = 10}
  VVI_Pace_Heart -> VVI_Charging_Discharging : after(pulse_width,msec) / {NextState = 8}
  data: ModeOn input; State output int8; ATR_CMP_DETECT input boolean; VENT_CMP_DETECT input; p_lowrateinterval input; PACE_CHARGE_CTRL output boolean; Z_ATR_CTRL output boolean; Z_VENT_CTRL output boolean; PACE_GND_CTRL output boolean; ATR_PACE_CTRL output boolean; ATR_GND_CTRL output boolean; VENT_GND_CTRL output boolean; pulse_width input; VENT_PACE_CTRL output boolean; refract_period input; FRONTEND_CTRL output boolean; NextState output int8; p_lowerateinterval input; StateTran output boolean
